simulink model "naolinear"  (R2019a)
settings: Solver=VariableStepAuto  StartTime=0.0  StopTime=10.0  RelTol=1e-3
values from neighbouring files (symbols this model uses):
  A = [0 0 1 0;0 0 0 1;k 0 0 x;0 k -x 0]    [autovalores.m]    (also in graficoim.m = 0.0004; sim1.m = [zeros(2) eye(2);Ke*eye(2) -Ge]; sim2.m = [zeros(2) eye(2);Ke*eye(2) -Ge])
  B = kb*[zeros(2);eye(2)]    [autovalores.m]    (also in sim1.m = (1/J)*d*b*ki*[zeros(2);eye(2)]; sim2.m = (1/J)*d*b*ki*[zeros(2);eye(2)])
  C = [eye(2) zeros(2)]    [autovalores.m]    (also in sim1.m; sim2.m)
  F = Fdn    [sim1.m]    (also in sim2.m)
  Ki = 200    [sim1.m]    (also in simu_naolinear.m)
  x0 = [0.0002;-0.0002;0;0]    [sim1.m]    (also in sim2.m)
settings Model: Creator=vinic  LastModifiedBy=vinic

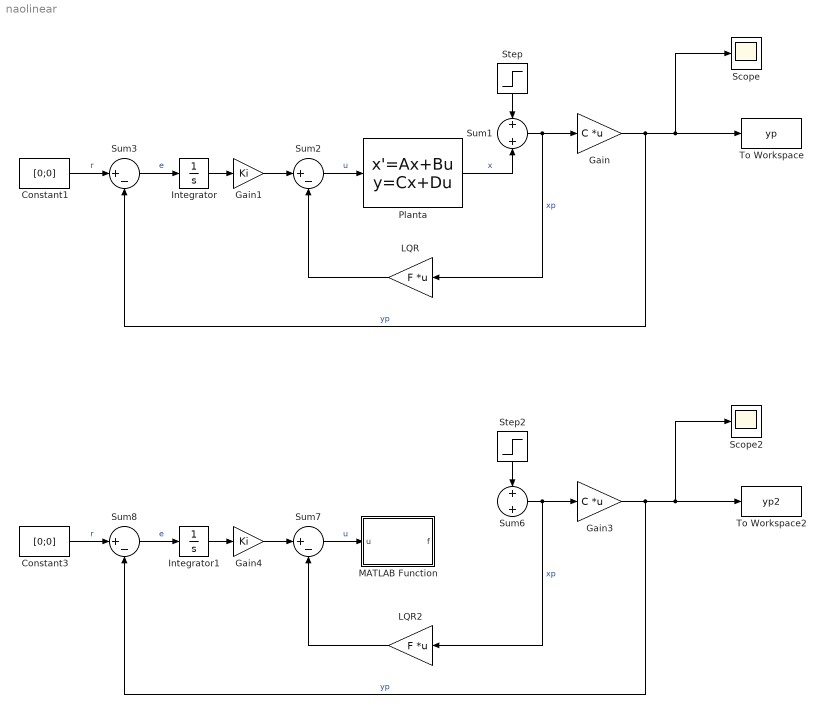
== system naolinear ==
  Constant1 : Constant  Value=[0;0]
  Constant3 : Constant  Value=[0;0]
  Gain : Gain  Gain=C  Multiplication=Matrix(K*u)
  Gain1 : Gain  Gain=Ki
  Gain3 : Gain  Gain=C  Multiplication=Matrix(K*u)
  Gain4 : Gain  Gain=Ki
  Integrator : Integrator
  Integrator1 : Integrator
  LQR : Gain  Gain=F  Multiplication=Matrix(K*u)
  LQR2 : Gain  Gain=F  Multiplication=Matrix(K*u)
  MATLAB Function : MATLAB Function  TreatAsAtomicUnit=on
  Planta : StateSpace  A=A  B=B  C=[eye(4)]  D=zeros(4,2)  InitialCondition=x0
  Scope : Scope
  Scope2 : Scope
  Step : Step  Time=0.5  After=[0.0002;-0.0002;0;0]  SampleTime=0
  Step2 : Step  Time=0.5  After=[0.0002;-0.0002;0;0]  SampleTime=0
  Sum1 : Sum
  Sum{2..3,7..8} (4 alike) : Sum  Inputs=|+-
  Sum6 : Sum
  To Workspace : ToWorkspace  VariableName=yp  SampleTime=-1
      settings: Save2DSignal=2-D array (concatenate along first dimension)
  To Workspace2 : ToWorkspace  VariableName=yp2  SampleTime=-1
      settings: Save2DSignal=2-D array (concatenate along first dimension)
  wires:
  Integrator1/1 -> Gain4/1
  Sum6/1 -> Gain3/1, LQR2/1  "xp"
  LQR2/1 -> Sum7/2
  Sum8/1 -> Integrator1/1  "e"
  Step2/1 -> Sum6/1
  Constant3/1 -> Sum8/1  "r"
  ? -> Sum6/2  "x"
  Constant1/1 -> Sum3/1  "r"
  Gain/1 -> Scope/1, To Workspace/1, Sum3/2  "yp"
  Gain1/1 -> Sum2/1
  Gain3/1 -> Scope2/1, To Workspace2/1, Sum8/2  "yp"
  Sum7/1 -> MATLAB Function/1(u)  "u"
  Sum3/1 -> Integrator/1  "e"
  Sum1/1 -> Gain/1, LQR/1  "xp"
  Step/1 -> Sum1/1
  Sum2/1 -> Planta/1  "u"
  Integrator/1 -> Gain1/1
  Planta/1 -> Sum1/2  "x"
  LQR/1 -> Sum2/2
  Gain4/1 -> Sum7/1

== matlab function naolinear/MATLAB Function ==
  data: u input; f output
function f = fcn(u)

i0 = 0.2325;
mu = 4*pi*10^(-7);
A = 4*10^(-4);
h = 0.5*10^(-3);
n = 300;
x = 0.2*10^(-3);
y = -0.2*10^(-3);


i1 = i0+id1;
i2 = i1;
i3 = id3;
u = [sqrt(3)/3*id3;id1];


R1 = (1/(mu *A))*(h-x*sqrt(3)/2-y/2);
R2 = (1/(mu *A))*(h+x*sqrt(3)/2-y/2);
R3 = (1/(mu *A))*(h+y);

N = R1*R2 + R1*R3 + R2*R3;
phi1 = (n/N)*((R2 + R3)*i1 + R3*i2 - R2*i3);
phi2 = (n/N)*(-R3*i1 -(R1+ R3)*i2 - R1*i3);
phi3 = (n/N)*(-R2*i1 +R1*i2 +(R1 + R2)*i3);

fx = sqrt(3)/(4 * mu * A)*(phi1^2 - phi2^2);
fy = 1/(4 * mu * A)*(phi1^2 + phi2^2 - phi3^2);


f = [fx;fy];
end
